simulink model "TEP_Final_NoScript"  (R2024a)
settings: Solver=FixedStepAuto  StartTime=0.0  StopTime=10  FixedStep=1/3600  RelTol=1e-3
model workspace (MAT data in the model file):
  AD : Simulink.Parameter (value not decoded)
  AG : Simulink.Parameter (value not decoded)
  AH : Simulink.Parameter (value not decoded)
  AV : Simulink.Parameter (value not decoded)
  AVP : Simulink.Parameter (value not decoded)
  BCHL : Simulink.Parameter (value not decoded)
  BCHV : Simulink.Parameter (value not decoded)
  BD : Simulink.Parameter (value not decoded)
  BG : Simulink.Parameter (value not decoded)
  BH : Simulink.Parameter (value not decoded)
  BVP : Simulink.Parameter (value not decoded)
  CD : Simulink.Parameter (value not decoded)
  CG : Simulink.Parameter (value not decoded)
  CH : Simulink.Parameter (value not decoded)
  CVP : Simulink.Parameter (value not decoded)
  XMW : Simulink.Parameter (value not decoded)
  XNS : Simulink.Parameter (value not decoded)
  XNSE : Simulink.Parameter (value not decoded)
symbols that are objects in the model workspace (value not decoded): AD, AG, AH, AV, AVP, BD, BG, BH, BVP, CD, CG, CH, CVP, XMW, XNS, XNSE
undefined symbols (not defined in the file or in its folder): magnitude, msgbox, SETPT, XMEAS, XMV
libraries: mylib x360, dspindex x28
(part 4 of 14)

== system TEP_Final_NoScript/Subsystem1/A feed stream ==
  Stream 3 : Inport
  Bus Creator : BusCreator  Inputs=4
  Bus Selector : BusSelector  OutputSignals=XMNSE(5),XMNSE(6)
  Bus Selector1 : BusSelector  OutputSignals=TST(3),XST(I;3)
  Bus Selector2 : BusSelector  OutputSignals=Stream 3
  Bus Selector3 : BusSelector  OutputSignals=signal1.XMEAS(1)
  Composition measurement mol% : Subsystem
  Constant : Constant  Value=1000
  Flow measurement in kg/h : Subsystem
  Pressure measurement in kPa : Subsystem
  Temperature measurement in C : Subsystem
  SMEAS 3 : Outport
  tag scope: SM3=global
  wires:
  Bus Selector1/1 -> Temperature measurement in C/1(T in celsius)  "<TST(3)>"
  Temperature measurement in C/1(SMEAST) -> Bus Creator/1
  [XMNSE] -> Bus Selector/1
  Bus Selector/1 -> Temperature measurement in C/2(XMNSE)  "<XMNSE(5)>"
  Bus Selector/2 -> Pressure measurement in kPa/2(XMNSE)  "<XMNSE(6)>"
  Stream 3/1 -> Bus Selector1/1
  Bus Selector1/2 -> Flow measurement in kg/h/2(XST), Composition measurement mol%/1(XST)  "<XST(I;3)>"
  Constant/1 -> Pressure measurement in kPa/1("P in mm Hg ")
  Pressure measurement in kPa/1(SMEASP) -> Bus Creator/2
  Flow measurement in kg/h/1("SMEASF ") -> Bus Creator/3  "SMEASF"
  Composition measurement mol%/1(SMEASX) -> Bus Creator/4
  Bus Creator/1 -> [SM3], SMEAS 3/1
  [XMNSE2] -> Bus Selector2/1
  Bus Selector2/1 -> Composition measurement mol%/2(XMNSE)  "<Stream 3>"
  [XMEAS] -> Bus Selector3/1
  Bus Selector3/1 -> Flow measurement in kg/h/1(XMEAS in kscmh)  "<XMEAS(1)>"

== system TEP_Final_NoScript/Subsystem1/CCIn ==
  Bus Creator : BusCreator  Inputs=3
  Bus Selector : BusSelector  OutputSignals=XMNSE(20),XMNSE(21),XMNSE(22)
  Flow measurement in kg/h : Subsystem
  Pressure measurement in kPa : Subsystem
  Temperature measurement in C : Subsystem
  SMEASCCWin : Outport
  tag scope: SMCC1=global
  wires:
  [TCWS] -> Pressure measurement in kPa/2(TC), Temperature measurement in C/1(T in celsius)
  Bus Creator/1 -> [SMCC1], SMEASCCWin/1
  [FWS] -> Flow measurement in kg/h/2(F in gpm)
  [XMNSE] -> Bus Selector/1
  Bus Selector/1 -> Temperature measurement in C/2(XMNSE)  "<XMNSE(20)>"
  Bus Selector/2 -> Pressure measurement in kPa/1(XMNSE)  "<XMNSE(21)>"
  Bus Selector/3 -> Flow measurement in kg/h/1(XMNSE)  "<XMNSE(22)>"
  Temperature measurement in C/1(SMEAST) -> Bus Creator/1
  Pressure measurement in kPa/1(SMEASP) -> Bus Creator/2
  Flow measurement in kg/h/1("SMEASF ") -> Bus Creator/3

== system TEP_Final_NoScript/Subsystem1/CCOut ==
  Bus Creator : BusCreator  Inputs=2
  Bus Selector : BusSelector  OutputSignals=XMNSE(23),XMNSE(24)
  Pressure measurement in kPa : Subsystem
  Temperature measurement in C : Subsystem
  SMEASCCWout : Outport
  tag scope: SMCC2=global
  wires:
  [TWS] -> Pressure measurement in kPa/2(TC), Temperature measurement in C/1(T in celsius)
  Bus Creator/1 -> [SMCC2], SMEASCCWout/1
  [XMNSE] -> Bus Selector/1
  Bus Selector/1 -> Temperature measurement in C/2(XMNSE)  "<XMNSE(23)>"
  Bus Selector/2 -> Pressure measurement in kPa/1(XMNSE)  "<XMNSE(24)>"
  Temperature measurement in C/1(SMEAST) -> Bus Creator/1
  Pressure measurement in kPa/1(SMEASP) -> Bus Creator/2

== system TEP_Final_NoScript/Subsystem1/CCin ==
  SMEAS : Inport
  Bus Selector : BusSelector  OutputSignals=SMEAST,SMEASP,SMEASF
  Subsystem : Subsystem
  Subsystem1 : Subsystem
  Subsystem3 : Subsystem
  tag scope: BMCC1=global, QS1=global
  wires:
  Bus Selector/1 -> Subsystem1/1(T), Subsystem3/1(TC)  "<SMEAST>"
  Subsystem/1(Bphm J/s) -> [BMCC1]  "BphmCC1"
  Subsystem3/1(Bph) -> Subsystem/1(Bph)  "BphRC1"
  Bus Selector/3 -> Subsystem1/2(F), Subsystem/2(FWR in kg/h)  "<SMEASF>"
  Subsystem1/1(Q J/s) -> [QS1]
  Bus Selector/2 -> Subsystem3/2(P)  "<SMEASP>"
  SMEAS/1 -> Bus Selector/1

== system TEP_Final_NoScript/Subsystem1/CCout ==
  SMEAS : Inport
  SMEAS1 : Inport  Port=2
  Bus Selector : BusSelector  OutputSignals=SMEAST,SMEASP
  Bus Selector1 : BusSelector  OutputSignals=SMEASF
  Subsystem : Subsystem
  Subsystem1 : Subsystem
  Subsystem3 : Subsystem
  tag scope: BMCC2=global, QS2=global
  wires:
  Bus Selector/1 -> Subsystem3/1(TC), Subsystem1/1(T)  "<SMEAST>"
  Subsystem/1(Bphm J/s) -> [BMCC2]  "BphmCC2"
  Subsystem3/1(Bph) -> Subsystem/1(Bph)  "BphRC1"
  Bus Selector1/1 -> Subsystem1/2(F), Subsystem/2(FWR in kg/h)  "<SMEASF>"
  Subsystem1/1(Q J/s) -> [QS2]
  Bus Selector/2 -> Subsystem3/2(P)  "<SMEASP>"
  SMEAS/1 -> Bus Selector/1
  SMEAS1/1 -> Bus Selector1/1

== system TEP_Final_NoScript/Subsystem1/D feed stream ==
  Stream 1 : Inport
  Bus Creator : BusCreator  Inputs=4
  Bus Selector : BusSelector  OutputSignals=XMNSE(1),XMNSE(2)
  Bus Selector1 : BusSelector  OutputSignals=TST(1),XST(I;1)
  Bus Selector2 : BusSelector  OutputSignals=Stream 1
  Bus Selector3 : BusSelector  OutputSignals=signal1.XMEAS(2)
  Composition measurement mol% : Subsystem
  Constant : Constant  Value=1000
  Flow measurement in kg/h : Subsystem
  Pressure measurement in kPa : Subsystem
  Temperature measurement in C : Subsystem
  SMEAS 1 : Outport
  tag scope: SM1=global
  wires:
  Bus Selector1/1 -> Temperature measurement in C/1(T in celsius)  "<TST(1)>"
  Temperature measurement in C/1(SMEAST) -> Bus Creator/1
  [XMNSE] -> Bus Selector/1
  Bus Selector/1 -> Temperature measurement in C/2(XMNSE)  "<XMNSE(1)>"
  Bus Selector/2 -> Pressure measurement in kPa/2(XMNSE)  "<XMNSE(2)>"
  Stream 1/1 -> Bus Selector1/1
  Bus Selector1/2 -> Composition measurement mol%/1(XST)  "<XST(I;1)>"
  Constant/1 -> Pressure measurement in kPa/1("P in mm Hg ")
  Pressure measurement in kPa/1(SMEASP) -> Bus Creator/2
  Flow measurement in kg/h/1("SMEASF ") -> Bus Creator/3  "SMEASF"
  Composition measurement mol%/1(SMEASX) -> Bus Creator/4
  Bus Creator/1 -> [SM1], SMEAS 1/1
  [XMNSE2] -> Bus Selector2/1
  Bus Selector2/1 -> Composition measurement mol%/2(XMNSE)  "<Stream 1>"
  [XMEAS] -> Bus Selector3/1
  Bus Selector3/1 -> Flow measurement in kg/h/1(XMEAS in kg/h)  "<XMEAS(2)>"

== system TEP_Final_NoScript/Subsystem1/E feed stream ==
  Stream 2 : Inport
  Bus Creator : BusCreator  Inputs=4
  Bus Selector : BusSelector  OutputSignals=XMNSE(3),XMNSE(4)
  Bus Selector1 : BusSelector  OutputSignals=TST(2),XST(I;2)
  Bus Selector2 : BusSelector  OutputSignals=Stream 2
  Bus Selector3 : BusSelector  OutputSignals=signal1.XMEAS(3)
  Composition measurement mol% : Subsystem
  Constant : Constant  Value=1000
  Flow measurement in kg/h : Subsystem
  Pressure measurement in kPa : Subsystem
  Temperature measurement in C : Subsystem
  SMEAS 2 : Outport
  tag scope: SM2=global
  wires:
  Bus Selector1/1 -> Temperature measurement in C/1(T in celsius)  "<TST(2)>"
  Temperature measurement in C/1(SMEAST) -> Bus Creator/1
  [XMNSE] -> Bus Selector/1
  Bus Selector/1 -> Temperature measurement in C/2(XMNSE)  "<XMNSE(3)>"
  Bus Selector/2 -> Pressure measurement in kPa/2(XMNSE)  "<XMNSE(4)>"
  Stream 2/1 -> Bus Selector1/1
  Bus Selector1/2 -> Composition measurement mol%/1(XST)  "<XST(I;2)>"
  Constant/1 -> Pressure measurement in kPa/1("P in mm Hg ")
  Pressure measurement in kPa/1(SMEASP) -> Bus Creator/2
  Flow measurement in kg/h/1("SMEASF ") -> Bus Creator/3  "SMEASF"
  Composition measurement mol%/1(SMEASX) -> Bus Creator/4
  Bus Creator/1 -> [SM2], SMEAS 2/1
  [XMNSE2] -> Bus Selector2/1
  Bus Selector2/1 -> Composition measurement mol%/2(XMNSE)  "<Stream 2>"
  [XMEAS] -> Bus Selector3/1
  Bus Selector3/1 -> Flow measurement in kg/h/1(XMEAS in kg/h)  "<XMEAS(3)>"

== system TEP_Final_NoScript/Subsystem1/Product stream ==
  Stream 13 : Inport
  Bus Creator : BusCreator  Inputs=4
  Bus Selector : BusSelector  OutputSignals=XMNSE(14)
  Bus Selector1 : BusSelector  OutputSignals=PTC,XST(I;13)
  Bus Selector2 : BusSelector  OutputSignals=Stream 13
  Bus Selector3 : BusSelector  OutputSignals=signal4.XMEAS(18),signal4.XMEAS(17)
  Bus Selector4 : BusSelector  OutputSignals=Stream 13
  Composition measurement mol% : Subsystem
  Flow measurement in kg/h : Subsystem
  Pressure measurement in kPa : Subsystem
  Temperature measurement in C : Subsystem
  SMEAS 13 : Outport
  tag scope: SM13=global
  wires:
  Temperature measurement in C/1(SMEAST) -> Bus Creator/1
  [XMNSE] -> Bus Selector/1
  Stream 13/1 -> Bus Selector1/1
  Pressure measurement in kPa/1(SMEASP) -> Bus Creator/2
  Flow measurement in kg/h/1("SMEASF ") -> Bus Creator/3  "SMEASF"
  Composition measurement mol%/1(SMEASX) -> Bus Creator/4
  Bus Creator/1 -> [SM13], SMEAS 13/1
  [XMNSE2] -> Bus Selector2/1
  Bus Selector2/1 -> Composition measurement mol%/2(XMNSE2)  "<Stream 13>"
  [XMEAS] -> Bus Selector3/1
  Bus Selector/1 -> Pressure measurement in kPa/2(XMNSE)  "<XMNSE(14)>"
  Bus Selector1/1 -> Pressure measurement in kPa/1("P in mm Hg ")  "<PTC>"
  Bus Selector3/1 -> Temperature measurement in C/1(XMEAS in celsius)  "<XMEAS(18)>"
  Bus Selector3/2 -> Flow measurement in kg/h/1(XMEAS in m^3/h)  "<XMEAS(17)>"
  Bus Selector1/2 -> Composition measurement mol%/1(XST), Flow measurement in kg/h/2(XST)  "<XST(I;13)>"
  [XMNSE3] -> Bus Selector4/1
  Bus Selector4/1 -> Composition measurement mol%/3(XMNSE3)  "<Stream 13>"

== system TEP_Final_NoScript/Subsystem1/Purge stream ==
  Stream 10 : Inport
  Bus Creator : BusCreator  Inputs=4
  Bus Selector1 : BusSelector  OutputSignals=signal1.XST(I;10)
  Bus Selector3 : BusSelector  OutputSignals=signal3.XMEAS(11),signal3.XMEAS(13),signal3.XMEAS(10),signal9
  Composition measurement mol% : Subsystem
  Flow measurement in kg/h : Subsystem
  Pressure measurement in kPa : Subsystem
  Temperature measurement in C : Subsystem
  SMEAS 10 : Outport
  tag scope: SM10=global
  wires:
  Temperature measurement in C/1(SMEAST) -> Bus Creator/1  "SMEAST"
  Stream 10/1 -> Bus Selector1/1
  Bus Selector1/1 -> Flow measurement in kg/h/2(XST)  "<XST(I;10)>"
  Pressure measurement in kPa/1(SMEASP) -> Bus Creator/2
  Flow measurement in kg/h/1("SMEASF ") -> Bus Creator/3  "SMEASF"
  Composition measurement mol%/1(SMEASX) -> Bus Creator/4
  Bus Creator/1 -> [SM10], SMEAS 10/1
  [XMEAS] -> Bus Selector3/1
  Bus Selector3/1 -> Temperature measurement in C/1(XMEAS in celsius)  "<XMEAS(11)>"
  Bus Selector3/2 -> Pressure measurement in kPa/1(XMEAS in kPa gauge)  "<XMEAS(13)>"
  Bus Selector3/3 -> Flow measurement in kg/h/1(XMEAS in kscmh)  "<XMEAS(10)>"
  Bus Selector3/4 -> Composition measurement mol%/1(XMEAS)  "<signal9>"

== system TEP_Final_NoScript/Subsystem1/RCIn ==
  Bus Creator : BusCreator  Inputs=3
  Bus Selector : BusSelector  OutputSignals=XMNSE(15),XMNSE(16),XMNSE(17)
  Flow measurement in kg/h : Subsystem
  Pressure measurement in kPa : Subsystem
  Temperature measurement in C : Subsystem
  SMEASRCWin : Outport
  tag scope: SMRC1=global
  wires:
  [TCWR] -> Pressure measurement in kPa/2(TC), Temperature measurement in C/1(T in celsius)
  [FWR] -> Flow measurement in kg/h/2(F in gpm)
  [XMNSE] -> Bus Selector/1
  Bus Selector/1 -> Temperature measurement in C/2(XMNSE)  "<XMNSE(15)>"
  Bus Selector/2 -> Pressure measurement in kPa/1(XMNSE)  "<XMNSE(16)>"
  Bus Selector/3 -> Flow measurement in kg/h/1(XMNSE)  "<XMNSE(17)>"
  Temperature measurement in C/1(SMEAST) -> Bus Creator/1
  Pressure measurement in kPa/1(SMEASP) -> Bus Creator/2
  Flow measurement in kg/h/1("SMEASF ") -> Bus Creator/3
  Bus Creator/1 -> [SMRC1], SMEASRCWin/1

== system TEP_Final_NoScript/Subsystem1/RCOut ==
  Bus Creator : BusCreator  Inputs=2
  Bus Selector : BusSelector  OutputSignals=XMNSE(18),XMNSE(19)
  Pressure measurement in kPa : Subsystem
  Temperature measurement in C : Subsystem
  SMEASRCWout : Outport
  tag scope: SMRC2=global
  wires:
  [TWR] -> Pressure measurement in kPa/2(TC), Temperature measurement in C/1(T in celsius)
  Bus Creator/1 -> [SMRC2], SMEASRCWout/1
  [XMNSE] -> Bus Selector/1
  Bus Selector/1 -> Temperature measurement in C/2(XMNSE)  "<XMNSE(18)>"
  Bus Selector/2 -> Pressure measurement in kPa/1(XMNSE)  "<XMNSE(19)>"
  Temperature measurement in C/1(SMEAST) -> Bus Creator/1
  Pressure measurement in kPa/1(SMEASP) -> Bus Creator/2

== system TEP_Final_NoScript/Subsystem1/RCin ==
  SMEAS : Inport
  Bus Selector : BusSelector  OutputSignals=SMEAST,SMEASP,SMEASF
  Subsystem : Subsystem
  Subsystem1 : Subsystem
  Subsystem3 : Subsystem
  tag scope: BMRC1=global, QR1=global
  wires:
  Bus Selector/1 -> Subsystem1/1(T), Subsystem3/1(TC)  "<SMEAST>"
  Subsystem/1(Bphm J/s) -> [BMRC1]  "BphmRC1"
  Subsystem3/1(Bph) -> Subsystem/1(Bph)  "BphRC1"
  Bus Selector/3 -> Subsystem1/2(F), Subsystem/2(FWR in kg/h)  "<SMEASF>"
  Subsystem1/1(Q J/s) -> [QR1]
  Bus Selector/2 -> Subsystem3/2(P)  "<SMEASP>"
  SMEAS/1 -> Bus Selector/1

== system TEP_Final_NoScript/Subsystem1/RCout ==
  SMEAS : Inport
  SMEAS1 : Inport  Port=2
  Bus Selector : BusSelector  OutputSignals=SMEAST,SMEASP
  Bus Selector1 : BusSelector  OutputSignals=SMEASF
  Subsystem : Subsystem
  Subsystem1 : Subsystem
  Subsystem3 : Subsystem
  tag scope: BMRC2=global, QR2=global
  wires:
  Bus Selector/1 -> Subsystem3/1(TC), Subsystem1/1(T)  "<SMEAST>"
  Subsystem/1(Bphm J/s) -> [BMRC2]  "BphmRC2"
  Subsystem3/1(Bph) -> Subsystem/1(Bph)  "BphRC1"
  Bus Selector1/1 -> Subsystem1/2(F), Subsystem/2(FWR in kg/h)  "<SMEASF>"
  Subsystem1/1(Q J/s) -> [QR2]
  Bus Selector/2 -> Subsystem3/2(P)  "<SMEASP>"
  SMEAS/1 -> Bus Selector/1
  SMEAS1/1 -> Bus Selector1/1

== system TEP_Final_NoScript/Subsystem1/Reactor feed stream ==
  Stream 6 : Inport
  Bus Creator : BusCreator  Inputs=4
  Bus Selector : BusSelector  OutputSignals=XMNSE(11)
  Bus Selector1 : BusSelector  OutputSignals=signal1.TST(6) = TST(7),signal1.XST(I;6) = XST(I;7)
  Bus Selector2 : BusSelector  OutputSignals=Stream 6
  Bus Selector3 : BusSelector  OutputSignals=signal4.XMEAS(16),signal2.XMEAS(6),signal8
  Composition measurement mol% : Subsystem
  Flow measurement in kg/h : Subsystem
  Pressure measurement in kPa : Subsystem
  Temperature measurement in C : Subsystem
  SMEAS 6 : Outport
  tag scope: SM6=global
  wires:
  Bus Selector1/1 -> Temperature measurement in C/1(T in celsius)  "<TST(6) = TST(7)>"
  Temperature measurement in C/1(SMEAST) -> Bus Creator/1
  [XMNSE] -> Bus Selector/1
  Bus Selector/1 -> Temperature measurement in C/2(XMNSE)  "<XMNSE(11)>"
  Stream 6/1 -> Bus Selector1/1
  Bus Selector1/2 -> Flow measurement in kg/h/2(XST), Composition measurement mol%/1(XST)  "<XST(I;6) = XST(I;7)>"
  [XMEAS] -> Bus Selector3/1
  Pressure measurement in kPa/1(SMEASP) -> Bus Creator/2
  Flow measurement in kg/h/1("SMEASF ") -> Bus Creator/3  "SMEASF"
  Composition measurement mol%/1(SMEASX) -> Bus Creator/4
  Bus Creator/1 -> [SM6], SMEAS 6/1
  [XMNSE2] -> Bus Selector2/1
  Bus Selector2/1 -> Composition measurement mol%/2(XMNSE)  "<Stream 6>"
  Bus Selector3/1 -> Pressure measurement in kPa/1(XMEAS in kPa gauge)  "<XMEAS(16)>"
  Bus Selector3/2 -> Flow measurement in kg/h/1(XMEAS in kscmh)  "<XMEAS(6)>"
  Bus Selector3/3 -> Composition measurement mol%/3(XMEAS)  "<signal8>"

== system TEP_Final_NoScript/Subsystem1/Reactor product stream ==
  Stream 8 : Inport
  Bus Creator : BusCreator  Inputs=4
  Bus Selector : BusSelector  OutputSignals=XMNSE(12)
  Bus Selector1 : BusSelector  OutputSignals=signal1.XST(I;8),signal1.FTM(8)
  Bus Selector2 : BusSelector  OutputSignals=Stream 8
  Bus Selector3 : BusSelector  OutputSignals=signal2.XMEAS(9),signal2.XMEAS(7)
  Composition measurement mol% : Subsystem
  Flow measurement in kg/h : Subsystem
  Pressure measurement in kPa : Subsystem
  Temperature measurement in C : Subsystem
  SMEAS 8 : Outport
  tag scope: SM8=global
  wires:
  Temperature measurement in C/1(SMEAST) -> Bus Creator/1
  [XMNSE] -> Bus Selector/1
  Stream 8/1 -> Bus Selector1/1
  Bus Selector1/1 -> Composition measurement mol%/1(XST), Flow measurement in kg/h/1(XST)  "<XST(I;8)>"
  Pressure measurement in kPa/1(SMEASP) -> Bus Creator/2
  Flow measurement in kg/h/1("SMEASF ") -> Bus Creator/3
  Composition measurement mol%/1(SMEASX) -> Bus Creator/4
  Bus Creator/1 -> [SM8], SMEAS 8/1
  [XMNSE2] -> Bus Selector2/1
  Bus Selector2/1 -> Composition measurement mol%/2(XMNSE)  "<Stream 8>"
  [XMEAS] -> Bus Selector3/1
  Bus Selector3/1 -> Temperature measurement in C/1(XMEAS in celsius)  "<XMEAS(9)>"
  Bus Selector3/2 -> Pressure measurement in kPa/1(XMEAS in kPa gauge)  "<XMEAS(7)>"
  Bus Selector1/2 -> Flow measurement in kg/h/3(F in lb-mol/h)  "<FTM(8)>"
  Bus Selector/1 -> Flow measurement in kg/h/2(XMNSE)  "<XMNSE(12)>"

== system TEP_Final_NoScript/Subsystem1/Separator recycle stream ==
  Stream 9 : Inport
  Bus Creator : BusCreator  Inputs=4
  Bus Selector1 : BusSelector  OutputSignals=signal2.XST(I;9)
  Bus Selector2 : BusSelector  OutputSignals=Stream 9
  Bus Selector3 : BusSelector  OutputSignals=signal3.XMEAS(11),signal3.XMEAS(13),signal1.XMEAS(5)
  Composition measurement mol% : Subsystem
  Flow measurement in kg/h : Subsystem
  Pressure measurement in kPa : Subsystem
  Temperature measurement in C : Subsystem
  SMEAS 9 : Outport
  tag scope: SM9=global
  wires:
  Temperature measurement in C/1(SMEAST) -> Bus Creator/1  "SMEAST"
  Stream 9/1 -> Bus Selector1/1
  Bus Selector1/1 -> Flow measurement in kg/h/2(XST), Composition measurement mol%/1(XST)  "<XST(I;9)>"
  Pressure measurement in kPa/1(SMEASP) -> Bus Creator/2
  Flow measurement in kg/h/1("SMEASF ") -> Bus Creator/3  "SMEASF"
  Composition measurement mol%/1(SMEASX) -> Bus Creator/4
  Bus Creator/1 -> [SM9], SMEAS 9/1
  [XMNSE2] -> Bus Selector2/1
  Bus Selector2/1 -> Composition measurement mol%/2(XMNSE)  "<Stream 9>"
  [XMEAS] -> Bus Selector3/1
  Bus Selector3/1 -> Temperature measurement in C/1(XMEAS in celsius)  "<XMEAS(11)>"
  Bus Selector3/2 -> Pressure measurement in kPa/1(XMEAS in kPa gauge)  "<XMEAS(13)>"
  Bus Selector3/3 -> Flow measurement in kg/h/1(XMEAS in kscmh)  "<XMEAS(5)>"

== system TEP_Final_NoScript/Subsystem1/Separator underflow stream ==
  Stream 11 : Inport
  Bus Creator : BusCreator  Inputs=4
  Bus Selector1 : BusSelector  OutputSignals=signal1.PTSL,signal1.XST(I;11)
  Bus Selector2 : BusSelector  OutputSignals=Stream 11
  Bus Selector3 : BusSelector  OutputSignals=signal3.XMEAS(11),signal3.XMEAS(14)
  Bus Selector4 : BusSelector  OutputSignals=XMNSE(13)
  Composition measurement mol% : Subsystem
  Flow measurement in kg/h : Subsystem
  Pressure measurement in kPa : Subsystem
  Temperature measurement in C : Subsystem
  SMEAS 11 : Outport
  tag scope: SM11=global
  wires:
  Temperature measurement in C/1(SMEAST) -> Bus Creator/1
  [XMNSE] -> Bus Selector4/1
  Stream 11/1 -> Bus Selector1/1
  Pressure measurement in kPa/1(SMEASP) -> Bus Creator/2
  Flow measurement in kg/h/1("SMEASF ") -> Bus Creator/3  "SMEASF"
  Composition measurement mol%/1(SMEASX) -> Bus Creator/4
  Bus Creator/1 -> [SM11], SMEAS 11/1
  [XMNSE3] -> Bus Selector2/1
  Bus Selector2/1 -> Composition measurement mol%/2(XMNSE)  "<Stream 11>"
  [XMEAS] -> Bus Selector3/1
  Bus Selector4/1 -> Pressure measurement in kPa/2(XMNSE)  "<XMNSE(13)>"
  Bus Selector1/1 -> Pressure measurement in kPa/1("P in mm Hg ")  "<PTSL>"
  Bus Selector1/2 -> Flow measurement in kg/h/2(XST), Composition measurement mol%/1(XST)  "<XST(I;11)>"
  Bus Selector3/1 -> Temperature measurement in C/1(XMEAS in celsius)  "<XMEAS(11)>"
  Bus Selector3/2 -> Flow measurement in kg/h/1(XMEAS in m^3/h)  "<XMEAS(14)>"

== system TEP_Final_NoScript/Subsystem1/Stripper recycle stream ==
  Stream 5 : Inport
  Bus Creator : BusCreator  Inputs=4
  Bus Selector : BusSelector  OutputSignals=XMNSE(9),XMNSE(10)
  Bus Selector1 : BusSelector  OutputSignals=TST(5),XST(I;5),FTM(5)
  Bus Selector2 : BusSelector  OutputSignals=Stream 5
  Bus Selector3 : BusSelector  OutputSignals=signal4.XMEAS(16)
  Composition measurement mol% : Subsystem
  Flow measurement in kg/h : Subsystem
  Pressure measurement in kPa : Subsystem
  Temperature measurement in C : Subsystem
  SMEAS 5 : Outport
  tag scope: SM5=global
  wires:
  Bus Selector1/1 -> Temperature measurement in C/1(T in celsius)  "<TST(5)>"
  Temperature measurement in C/1(SMEAST) -> Bus Creator/1
  [XMNSE] -> Bus Selector/1
  Bus Selector/1 -> Temperature measurement in C/2(XMNSE)  "<XMNSE(9)>"
  Stream 5/1 -> Bus Selector1/1
  Bus Selector1/2 -> Composition measurement mol%/1(XST), Flow measurement in kg/h/1(XST)  "<XST(I;5)>"
  [XMEAS] -> Bus Selector3/1
  Pressure measurement in kPa/1(SMEASP) -> Bus Creator/2
  Flow measurement in kg/h/1("SMEASF ") -> Bus Creator/3
  Composition measurement mol%/1(SMEASX) -> Bus Creator/4
  Bus Creator/1 -> [SM5], SMEAS 5/1
  [XMNSE2] -> Bus Selector2/1
  Bus Selector2/1 -> Composition measurement mol%/2(XMNSE)  "<Stream 5>"
  Bus Selector3/1 -> Pressure measurement in kPa/1(XMEAS in kPa gauge)  "<XMEAS(16)>"
  Bus Selector1/3 -> Flow measurement in kg/h/3(F in lb-mol/h)  "<FTM(5)>"
  Bus Selector/2 -> Flow measurement in kg/h/2(XMNSE)  "<XMNSE(10)>"

== system TEP_Final_NoScript/Subsystem1/Subsystem1 ==
  SMEAS 8 : Inport
  Bus Creator3 : BusCreator  Inputs=2
  Bus Selector1 : BusSelector  OutputSignals=SMEAST,SMEASP,SMEASF,SMEASX
  Bus Selector2 : BusSelector  OutputSignals=signal1.HST(8),signal1.Phase
  Exergy1 : mylib/Exergy  SystemSampleTime=-1  VariantActivationTime=update diagram  AllowFlexibleInterface=on  Latency=0  AutoFrameSizeCalculation=off
      settings: SourceProductName=TEP Library
  J/s : Gain  Gain=0.29307107e6
  Subsystem : mylib/Subsystem  SystemSampleTime=-1  VariantActivationTime=update diagram  AllowFlexibleInterface=on  Latency=0  AutoFrameSizeCalculation=off
      settings: SourceProductName=TEP Library
  Subsystem1 : Subsystem
  mmBtu/hr : Product
  tag scope: BM8=global, Q8=global
  wires:
  Exergy1/1 -> Subsystem/1  "Bch8"
  Exergy1/2 -> Subsystem/2  "Bph8"
  Subsystem/1 -> Bus Creator3/1  "Bchm8"
  Subsystem/2 -> Bus Creator3/2  "Bphm8"
  Bus Creator3/1 -> [BM8]  "BM8"
  mmBtu/hr/1 -> J/s/1
  J/s/1 -> [Q8]
  [PropertiesStream8] -> Bus Selector2/1
  SMEAS 8/1 -> Subsystem1/1(SMEASX)
  Subsystem1/1(SMEASXOut) -> Bus Selector1/1
  Bus Selector2/1 -> mmBtu/hr/2  "<HST(8)>"
  Bus Selector2/2 -> Exergy1/1  "<Phase>"
  Bus Selector1/1 -> Exergy1/2  "<SMEAST>"
  Bus Selector1/2 -> Exergy1/4  "<SMEASP>"
  Bus Selector1/3 -> mmBtu/hr/1, Subsystem/3  "<SMEASF>"
  Bus Selector1/4 -> Exergy1/3  "<SMEASX>"

== system TEP_Final_NoScript/Subsystem1/Subsystem10 ==
  Bus Creator : BusCreator  Inputs=15
  B : Outport  VectorParamsAs1DForOutWhenUnconnected=off
  wires:
  Bus Creator/1 -> B/1
  [BMCC1] -> Bus Creator/14
  [BM11] -> Bus Creator/10
  [BM5] -> Bus Creator/5
  [BM1] -> Bus Creator/1
  [BM6] -> Bus Creator/6
  [BM9] -> Bus Creator/8
  [BM3] -> Bus Creator/3
  [BM4] -> Bus Creator/4
  [BM10] -> Bus Creator/9
  [BMRC1] -> Bus Creator/12
  [BM2] -> Bus Creator/2
  [BM13] -> Bus Creator/11
  [BM8] -> Bus Creator/7
  [BMRC2] -> Bus Creator/13
  [BMCC2] -> Bus Creator/15

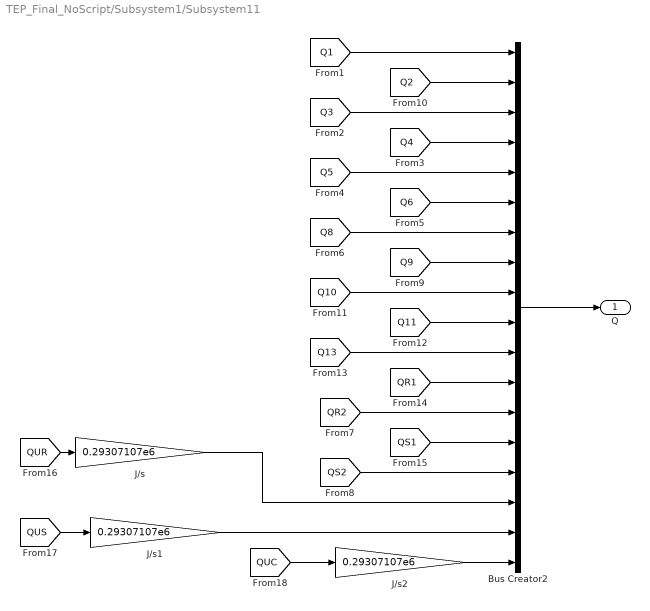
== system TEP_Final_NoScript/Subsystem1/Subsystem11 ==
  Bus Creator2 : BusCreator  Inputs=18
  J/s : Gain  Gain=0.29307107e6
  J/s1 : Gain  Gain=0.29307107e6
  J/s2 : Gain  Gain=0.29307107e6
  Q : Outport  VectorParamsAs1DForOutWhenUnconnected=off
  wires:
  [Q3] -> Bus Creator2/3
  Bus Creator2/1 -> Q/1
  [Q6] -> Bus Creator2/6
  [Q1] -> Bus Creator2/1
  [Q2] -> Bus Creator2/2
  [Q8] -> Bus Creator2/7
  [Q4] -> Bus Creator2/4
  [Q5] -> Bus Creator2/5
  [Q9] -> Bus Creator2/8
  [Q10] -> Bus Creator2/9
  [Q11] -> Bus Creator2/10
  [Q13] -> Bus Creator2/11
  [QR2] -> Bus Creator2/13
  [QR1] -> Bus Creator2/12
  [QS2] -> Bus Creator2/15
  [QS1] -> Bus Creator2/14
  [QUR] -> J/s/1
  J/s/1 -> Bus Creator2/16
  [QUS] -> J/s1/1
  J/s1/1 -> Bus Creator2/17
  [QUC] -> J/s2/1
  J/s2/1 -> Bus Creator2/18

== system TEP_Final_NoScript/Subsystem1/Subsystem13 ==
  SMEAS 6 : Inport
  Bus Creator3 : BusCreator  Inputs=2
  Bus Selector1 : BusSelector  OutputSignals=SMEAST,SMEASP,SMEASF,SMEASX
  Bus Selector2 : BusSelector  OutputSignals=signal1.HST(6) = HST(7),signal1.Phase
  Exergy1 : mylib/Exergy  SystemSampleTime=-1  VariantActivationTime=update diagram  AllowFlexibleInterface=on  Latency=0  AutoFrameSizeCalculation=off
      settings: SourceProductName=TEP Library
  J/s : Gain  Gain=0.29307107e6
  Subsystem : mylib/Subsystem  SystemSampleTime=-1  VariantActivationTime=update diagram  AllowFlexibleInterface=on  Latency=0  AutoFrameSizeCalculation=off
      settings: SourceProductName=TEP Library
  Subsystem1 : Subsystem
  mmBtu/hr : Product
  tag scope: BM6=global, Q6=global
  wires:
  Exergy1/1 -> Subsystem/1  "Bch6"
  Exergy1/2 -> Subsystem/2  "Bph6"
  Subsystem/1 -> Bus Creator3/1  "Bchm6"
  Subsystem/2 -> Bus Creator3/2  "Bphm6"
  Bus Creator3/1 -> [BM6]  "BM6"
  mmBtu/hr/1 -> J/s/1
  J/s/1 -> [Q6]
  SMEAS 6/1 -> Subsystem1/1(SMEASX)
  [PropertiesStream6] -> Bus Selector2/1
  Subsystem1/1(SMEASXOut) -> Bus Selector1/1
  Bus Selector2/1 -> mmBtu/hr/2  "<HST(6) = HST(7)>"
  Bus Selector2/2 -> Exergy1/1  "<Phase>"
  Bus Selector1/1 -> Exergy1/2  "<SMEAST>"
  Bus Selector1/2 -> Exergy1/4  "<SMEASP>"
  Bus Selector1/3 -> mmBtu/hr/1, Subsystem/3  "<SMEASF>"
  Bus Selector1/4 -> Exergy1/3  "<SMEASX>"

== system TEP_Final_NoScript/Subsystem1/Subsystem14 ==
  SMEAS 11 : Inport
  Bus Creator3 : BusCreator  Inputs=2
  Bus Selector1 : BusSelector  OutputSignals=SMEAST,SMEASP,SMEASF,SMEASX
  Bus Selector2 : BusSelector  OutputSignals=signal1.HST(11),signal1.Phase
  Exergy1 : mylib/Exergy  SystemSampleTime=-1  VariantActivationTime=update diagram  AllowFlexibleInterface=on  Latency=0  AutoFrameSizeCalculation=off
      settings: SourceProductName=TEP Library
  J/s : Gain  Gain=0.29307107e6
  Subsystem : mylib/Subsystem  SystemSampleTime=-1  VariantActivationTime=update diagram  AllowFlexibleInterface=on  Latency=0  AutoFrameSizeCalculation=off
      settings: SourceProductName=TEP Library
  Subsystem1 : Subsystem
  mmBtu/hr : Product
  tag scope: BM11=global, Q11=global
  wires:
  Exergy1/1 -> Subsystem/1  "Bch11"
  Exergy1/2 -> Subsystem/2  "Bph11"
  Subsystem/1 -> Bus Creator3/1  "Bchm11"
  Subsystem/2 -> Bus Creator3/2  "Bphm11"
  Bus Creator3/1 -> [BM11]  "BM11"
  J/s/1 -> [Q11]
  mmBtu/hr/1 -> J/s/1
  [PropertiesStream11] -> Bus Selector2/1
  SMEAS 11/1 -> Subsystem1/1(SMEASX)
  Subsystem1/1(SMEASXOut) -> Bus Selector1/1
  Bus Selector2/1 -> mmBtu/hr/2  "<HST(11)>"
  Bus Selector2/2 -> Exergy1/1  "<Phase>"
  Bus Selector1/1 -> Exergy1/2  "<SMEAST>"
  Bus Selector1/2 -> Exergy1/4  "<SMEASP>"
  Bus Selector1/3 -> Subsystem/3, mmBtu/hr/1  "<SMEASF>"
  Bus Selector1/4 -> Exergy1/3  "<SMEASX>"

== system TEP_Final_NoScript/Subsystem1/Subsystem15 ==
  SMEAS 2 : Inport
  Bus Creator3 : BusCreator  Inputs=2
  Bus Selector1 : BusSelector  OutputSignals=SMEAST,SMEASP,SMEASF,SMEASX
  Bus Selector2 : BusSelector  OutputSignals=HST(2)
  Exergy1 : mylib/Exergy  SystemSampleTime=-1  VariantActivationTime=update diagram  AllowFlexibleInterface=on  Latency=0  AutoFrameSizeCalculation=off
      settings: SourceProductName=TEP Library
  ITY : Constant
  J/s : Gain  Gain=0.29307107e6
  Subsystem : mylib/Subsystem  SystemSampleTime=-1  VariantActivationTime=update diagram  AllowFlexibleInterface=on  Latency=0  AutoFrameSizeCalculation=off
      settings: SourceProductName=TEP Library
  Subsystem1 : Subsystem
  mmBtu/hr : Product
  tag scope: BM2=global, Q2=global
  wires:
  Exergy1/1 -> Subsystem/1  "Bch2"
  Exergy1/2 -> Subsystem/2  "Bph2"
  Subsystem/1 -> Bus Creator3/1  "Bchm2"
  Subsystem/2 -> Bus Creator3/2  "Bphm2"
  Bus Creator3/1 -> [BM2]  "BM2"
  ITY/1 -> Exergy1/1
  mmBtu/hr/1 -> J/s/1
  J/s/1 -> [Q2]
  SMEAS 2/1 -> Subsystem1/1(SMEASX)
  Subsystem1/1(SMEASXOut) -> Bus Selector1/1
  Bus Selector1/1 -> Exergy1/2  "<SMEAST>"
  Bus Selector1/2 -> Exergy1/4  "<SMEASP>"
  Bus Selector1/3 -> Subsystem/3, mmBtu/hr/1  "<SMEASF>"
  Bus Selector1/4 -> Exergy1/3  "<SMEASX>"
  [PropertiesStream2] -> Bus Selector2/1
  Bus Selector2/1 -> mmBtu/hr/2  "<HST(2)>"

== system TEP_Final_NoScript/Subsystem1/Subsystem16 ==
  SMEAS 3 : Inport
  Bus Creator3 : BusCreator  Inputs=2
  Bus Selector1 : BusSelector  OutputSignals=SMEAST,SMEASP,SMEASF,SMEASX
  Bus Selector2 : BusSelector  OutputSignals=HST(3)
  Exergy1 : mylib/Exergy  SystemSampleTime=-1  VariantActivationTime=update diagram  AllowFlexibleInterface=on  Latency=0  AutoFrameSizeCalculation=off
      settings: SourceProductName=TEP Library
  ITY : Constant
  J/s : Gain  Gain=0.29307107e6
  Subsystem : mylib/Subsystem  SystemSampleTime=-1  VariantActivationTime=update diagram  AllowFlexibleInterface=on  Latency=0  AutoFrameSizeCalculation=off
      settings: SourceProductName=TEP Library
  Subsystem1 : Subsystem
  mmBtu/hr : Product
  tag scope: BM3=global, Q3=global
  wires:
  Exergy1/1 -> Subsystem/1  "Bch3"
  Exergy1/2 -> Subsystem/2  "Bph3"
  Subsystem/1 -> Bus Creator3/1  "Bchm3"
  Subsystem/2 -> Bus Creator3/2  "Bphm3"
  Bus Creator3/1 -> [BM3]  "BM3"
  ITY/1 -> Exergy1/1
  mmBtu/hr/1 -> J/s/1
  J/s/1 -> [Q3]
  Subsystem1/1(SMEASXOut) -> Bus Selector1/1
  SMEAS 3/1 -> Subsystem1/1(SMEASX)
  [PropertiesStream3] -> Bus Selector2/1
  Bus Selector2/1 -> mmBtu/hr/2  "<HST(3)>"
  Bus Selector1/1 -> Exergy1/2  "<SMEAST>"
  Bus Selector1/2 -> Exergy1/4  "<SMEASP>"
  Bus Selector1/3 -> Subsystem/3, mmBtu/hr/1  "<SMEASF>"
  Bus Selector1/4 -> Exergy1/3  "<SMEASX>"

== system TEP_Final_NoScript/Subsystem1/Subsystem17 ==
  SMEAS 4 : Inport
  Bus Creator3 : BusCreator  Inputs=2
  Bus Selector1 : BusSelector  OutputSignals=SMEAST,SMEASP,SMEASF,SMEASX
  Bus Selector2 : BusSelector  OutputSignals=HST(4)
  Exergy1 : mylib/Exergy  SystemSampleTime=-1  VariantActivationTime=update diagram  AllowFlexibleInterface=on  Latency=0  AutoFrameSizeCalculation=off
      settings: SourceProductName=TEP Library
  ITY : Constant
  J/s : Gain  Gain=0.29307107e6
  Subsystem : mylib/Subsystem  SystemSampleTime=-1  VariantActivationTime=update diagram  AllowFlexibleInterface=on  Latency=0  AutoFrameSizeCalculation=off
      settings: SourceProductName=TEP Library
  Subsystem1 : Subsystem
  mmBtu/hr : Product
  tag scope: BM4=global, Q4=global
  wires:
  Exergy1/1 -> Subsystem/1  "Bch4"
  Exergy1/2 -> Subsystem/2  "Bph4"
  Subsystem/1 -> Bus Creator3/1  "Bchm4"
  Subsystem/2 -> Bus Creator3/2  "Bphm4"
  Bus Creator3/1 -> [BM4]  "BM4"
  ITY/1 -> Exergy1/1
  mmBtu/hr/1 -> J/s/1
  J/s/1 -> [Q4]
  SMEAS 4/1 -> Subsystem1/1(SMEASX)
  [PropertiesStream4] -> Bus Selector2/1
  Subsystem1/1(SMEASXOut) -> Bus Selector1/1
  Bus Selector1/1 -> Exergy1/2  "<SMEAST>"
  Bus Selector1/2 -> Exergy1/4  "<SMEASP>"
  Bus Selector1/3 -> mmBtu/hr/1, Subsystem/3  "<SMEASF>"
  Bus Selector1/4 -> Exergy1/3  "<SMEASX>"
  Bus Selector2/1 -> mmBtu/hr/2  "<HST(4)>"

== system TEP_Final_NoScript/Subsystem1/Subsystem2 ==
  SMEAS 9 : Inport
  Bus Creator3 : BusCreator  Inputs=2
  Bus Selector1 : BusSelector  OutputSignals=SMEAST,SMEASP,SMEASF,SMEASX
  Bus Selector2 : BusSelector  OutputSignals=signal2.HST(9),signal2.Phase
  Exergy1 : mylib/Exergy  SystemSampleTime=-1  VariantActivationTime=update diagram  AllowFlexibleInterface=on  Latency=0  AutoFrameSizeCalculation=off
      settings: SourceProductName=TEP Library
  J/s : Gain  Gain=0.29307107e6
  Subsystem : mylib/Subsystem  SystemSampleTime=-1  VariantActivationTime=update diagram  AllowFlexibleInterface=on  Latency=0  AutoFrameSizeCalculation=off
      settings: SourceProductName=TEP Library
  Subsystem1 : Subsystem
  mmBtu/hr : Product
  tag scope: BM9=global, Q9=global
  wires:
  Exergy1/1 -> Subsystem/1  "Bch9"
  Exergy1/2 -> Subsystem/2  "Bph9"
  Subsystem/1 -> Bus Creator3/1  "Bchm9"
  Subsystem/2 -> Bus Creator3/2  "Bphm9"
  Bus Creator3/1 -> [BM9]  "BM9"
  mmBtu/hr/1 -> J/s/1
  J/s/1 -> [Q9]
  [PropertiesStream9] -> Bus Selector2/1
  SMEAS 9/1 -> Subsystem1/1(SMEASX)
  Subsystem1/1(SMEASXOut) -> Bus Selector1/1
  Bus Selector2/1 -> mmBtu/hr/2  "<HST(9)>"
  Bus Selector2/2 -> Exergy1/1  "<Phase>"
  Bus Selector1/1 -> Exergy1/2  "<SMEAST>"
  Bus Selector1/2 -> Exergy1/4  "<SMEASP>"
  Bus Selector1/3 -> mmBtu/hr/1, Subsystem/3  "<SMEASF>"
  Bus Selector1/4 -> Exergy1/3  "<SMEASX>"

== system TEP_Final_NoScript/Subsystem1/Subsystem3 ==
  SMEAS 10 : Inport
  Bus Creator3 : BusCreator  Inputs=2
  Bus Selector1 : BusSelector  OutputSignals=SMEAST,SMEASP,SMEASF,SMEASX
  Bus Selector2 : BusSelector  OutputSignals=signal1.HST(10),signal1.Phase
  Exergy1 : mylib/Exergy  SystemSampleTime=-1  VariantActivationTime=update diagram  AllowFlexibleInterface=on  Latency=0  AutoFrameSizeCalculation=off
      settings: SourceProductName=TEP Library
  J/s : Gain  Gain=0.29307107e6
  Subsystem : mylib/Subsystem  SystemSampleTime=-1  VariantActivationTime=update diagram  AllowFlexibleInterface=on  Latency=0  AutoFrameSizeCalculation=off
      settings: SourceProductName=TEP Library
  Subsystem1 : Subsystem
  mmBtu/hr : Product
  tag scope: BM10=global, Q10=global
  wires:
  Exergy1/1 -> Subsystem/1  "Bch10"
  Exergy1/2 -> Subsystem/2  "Bph10"
  Subsystem/1 -> Bus Creator3/1  "Bchm10"
  Subsystem/2 -> Bus Creator3/2  "Bphm10"
  Bus Creator3/1 -> [BM10]  "BM10"
  mmBtu/hr/1 -> J/s/1
  J/s/1 -> [Q10]
  [PropertiesStream10] -> Bus Selector2/1
  SMEAS 10/1 -> Subsystem1/1(SMEASX)
  Subsystem1/1(SMEASXOut) -> Bus Selector1/1
  Bus Selector2/1 -> mmBtu/hr/2  "<HST(10)>"
  Bus Selector2/2 -> Exergy1/1  "<Phase>"
  Bus Selector1/1 -> Exergy1/2  "<SMEAST>"
  Bus Selector1/2 -> Exergy1/4  "<SMEASP>"
  Bus Selector1/3 -> mmBtu/hr/1, Subsystem/3  "<SMEASF>"
  Bus Selector1/4 -> Exergy1/3  "<SMEASX>"

== system TEP_Final_NoScript/Subsystem1/Subsystem4 ==
  SMEAS 5 : Inport
  Bus Creator3 : BusCreator  Inputs=2
  Bus Selector1 : BusSelector  OutputSignals=SMEAST,SMEASP,SMEASF,SMEASX
  Bus Selector2 : BusSelector  OutputSignals=HST(5),Phase
  Exergy1 : mylib/Exergy  SystemSampleTime=-1  VariantActivationTime=update diagram  AllowFlexibleInterface=on  Latency=0  AutoFrameSizeCalculation=off
      settings: SourceProductName=TEP Library
  J/s : Gain  Gain=0.29307107e6
  Subsystem : mylib/Subsystem  SystemSampleTime=-1  VariantActivationTime=update diagram  AllowFlexibleInterface=on  Latency=0  AutoFrameSizeCalculation=off
      settings: SourceProductName=TEP Library
  Subsystem1 : Subsystem
  mmBtu/hr : Product
  tag scope: BM5=global, Q5=global
  wires:
  Exergy1/1 -> Subsystem/1  "Bch5"
  Exergy1/2 -> Subsystem/2  "Bph5"
  Subsystem/1 -> Bus Creator3/1  "Bchm5"
  Subsystem/2 -> Bus Creator3/2  "Bphm5"
  Bus Creator3/1 -> [BM5]  "BM5"
  J/s/1 -> [Q5]
  mmBtu/hr/1 -> J/s/1
  SMEAS 5/1 -> Subsystem1/1(SMEASX)
  [PropertiesStream5] -> Bus Selector2/1
  Subsystem1/1(SMEASXOut) -> Bus Selector1/1
  Bus Selector2/1 -> mmBtu/hr/2  "<HST(5)>"
  Bus Selector2/2 -> Exergy1/1  "<Phase>"
  Bus Selector1/1 -> Exergy1/2  "<SMEAST>"
  Bus Selector1/2 -> Exergy1/4  "<SMEASP>"
  Bus Selector1/3 -> Subsystem/3, mmBtu/hr/1  "<SMEASF>"
  Bus Selector1/4 -> Exergy1/3  "<SMEASX>"

== system TEP_Final_NoScript/Subsystem1/Subsystem5 ==
  SMEAS 13 : Inport
  Bus Creator3 : BusCreator  Inputs=2
  Bus Selector1 : BusSelector  OutputSignals=SMEAST,SMEASP,SMEASF,SMEASX
  Bus Selector2 : BusSelector  OutputSignals=HST(13),Phase
  Exergy1 : mylib/Exergy  SystemSampleTime=-1  VariantActivationTime=update diagram  AllowFlexibleInterface=on  Latency=0  AutoFrameSizeCalculation=off
      settings: SourceProductName=TEP Library
  J/s : Gain  Gain=0.29307107e6
  Subsystem : mylib/Subsystem  SystemSampleTime=-1  VariantActivationTime=update diagram  AllowFlexibleInterface=on  Latency=0  AutoFrameSizeCalculation=off
      settings: SourceProductName=TEP Library
  Subsystem1 : Subsystem
  mmBtu/hr : Product
  tag scope: BM13=global, Q13=global
  wires:
  Exergy1/1 -> Subsystem/1  "Bch13"
  Exergy1/2 -> Subsystem/2  "Bph13"
  Subsystem/1 -> Bus Creator3/1  "Bchm13"
  Subsystem/2 -> Bus Creator3/2  "Bphm13"
  Bus Creator3/1 -> [BM13]  "BM13"
  J/s/1 -> [Q13]
  mmBtu/hr/1 -> J/s/1
  [PropertiesStream13] -> Bus Selector2/1
  SMEAS 13/1 -> Subsystem1/1(SMEASX)
  Subsystem1/1(SMEASXOut) -> Bus Selector1/1
  Bus Selector2/1 -> mmBtu/hr/2  "<HST(13)>"
  Bus Selector2/2 -> Exergy1/1  "<Phase>"
  Bus Selector1/1 -> Exergy1/2  "<SMEAST>"
  Bus Selector1/2 -> Exergy1/4  "<SMEASP>"
  Bus Selector1/3 -> Subsystem/3, mmBtu/hr/1  "<SMEASF>"
  Bus Selector1/4 -> Exergy1/3  "<SMEASX>"

== system TEP_Final_NoScript/Subsystem1/Subsystem6 ==
  Bus Creator : BusCreator  Inputs=15
  SM : Outport  VectorParamsAs1DForOutWhenUnconnected=off
  wires:
  Bus Creator/1 -> SM/1
  [SMCC1] -> Bus Creator/14
  [SM11] -> Bus Creator/10
  [SM5] -> Bus Creator/5
  [SM1] -> Bus Creator/1
  [SM6] -> Bus Creator/6
  [SM9] -> Bus Creator/8
  [SM3] -> Bus Creator/3
  [SM4] -> Bus Creator/4
  [SM10] -> Bus Creator/9
  [SMRC1] -> Bus Creator/12
  [SM2] -> Bus Creator/2
  [SM13] -> Bus Creator/11
  [SM8] -> Bus Creator/7
  [SMRC2] -> Bus Creator/13
  [SMCC2] -> Bus Creator/15

== system TEP_Final_NoScript/Subsystem1/Subsystem8 ==
  SMEAS 1 : Inport
  Bus Creator3 : BusCreator  Inputs=2
  Bus Selector1 : BusSelector  OutputSignals=SMEAST,SMEASP,SMEASF,SMEASX
  Bus Selector2 : BusSelector  OutputSignals=HST(1)
  Exergy1 : mylib/Exergy  SystemSampleTime=-1  VariantActivationTime=update diagram  AllowFlexibleInterface=on  Latency=0  AutoFrameSizeCalculation=off
      settings: SourceProductName=TEP Library
  ITY : Constant
  J/s : Gain  Gain=0.29307107e6
  Subsystem : mylib/Subsystem  SystemSampleTime=-1  VariantActivationTime=update diagram  AllowFlexibleInterface=on  Latency=0  AutoFrameSizeCalculation=off
      settings: SourceProductName=TEP Library
  Subsystem1 : Subsystem
  mmBtu/hr : Product
  tag scope: BM1=global, Q1=global
  wires:
  Exergy1/1 -> Subsystem/1  "Bch1"
  Exergy1/2 -> Subsystem/2  "Bph1"
  Subsystem/1 -> Bus Creator3/1  "Bchm1"
  Subsystem/2 -> Bus Creator3/2  "Bphm1"
  Bus Creator3/1 -> [BM1]  "BM1"
  ITY/1 -> Exergy1/1
  J/s/1 -> [Q1]
  mmBtu/hr/1 -> J/s/1
  SMEAS 1/1 -> Subsystem1/1(SMEASX)
  [PropertiesStream1] -> Bus Selector2/1
  Subsystem1/1(SMEASXOut) -> Bus Selector1/1
  Bus Selector1/1 -> Exergy1/2  "<SMEAST>"
  Bus Selector1/2 -> Exergy1/4  "<SMEASP>"
  Bus Selector1/3 -> mmBtu/hr/1, Subsystem/3  "<SMEASF>"
  Bus Selector1/4 -> Exergy1/3  "<SMEASX>"
  Bus Selector2/1 -> mmBtu/hr/2  "<HST(1)>"

== system TEP_Final_NoScript/Valve/FTM(1) Total molar flow of Stream 1 lb-mol//h ==
  VPOS(1) : Inport
  VRNG(1) : Inport  Port=2
  " " : Product  Inputs=**/
  Constant : Constant  Value=100
  FTM(1) : Outport  PortDimensions=1  VectorParamsAs1DForOutWhenUnconnected=off
  wires:
  VRNG(1)/1 -> " "/2
  Constant/1 -> " "/3
  VPOS(1)/1 -> " "/1
  " "/1 -> FTM(1)/1

== system TEP_Final_NoScript/Valve/Position of Valve 1 % ==
  Bus Selector : BusSelector  OutputSignals=XMV(1)
  Control valve : mylib/Control valve  SystemSampleTime=-1  VariantActivationTime=update diagram  AllowFlexibleInterface=on  Latency=0  AutoFrameSizeCalculation=off
      settings: SourceProductName=TEP Library
  Display : Display
  Divide : Product  Inputs=*/
  IVST(1) : Constant  Value=0
  Integration : mylib/Integration  SystemSampleTime=-1  VariantActivationTime=update diagram  AllowFlexibleInterface=on  Latency=0  AutoFrameSizeCalculation=off
      settings: SourceProductName=TEP Library
  Subtract : Sum  Inputs=+-
  VTAU(1) : Constant  Value=8/3600
  YY(39) : Constant  Value=63.05263039
  "YY(39) " : Outport  VectorParamsAs1DForOutWhenUnconnected=off
  wires:
  Integration/1 -> "YY(39) "/1, Subtract/2  "VPOS(1)"
  YY(39)/1 -> Integration/2
  Subtract/1 -> Divide/1
  VTAU(1)/1 -> Divide/2
  Divide/1 -> Display/1, Integration/1
  Control valve/1 -> Subtract/1
  [XMV] -> Bus Selector/1
  Bus Selector/1 -> Control valve/1  "<XMV(1)>"
  IVST(1)/1 -> Control valve/2

== system TEP_Final_NoScript/Valve 2/FTM(2) Total molar flow of Stream 2 lb-mol//h ==
  VPOS(2) : Inport
  VRNG(2) : Inport  Port=2
  " " : Product  Inputs=**/
  Constant : Constant  Value=100
  FTM(2) : Outport  PortDimensions=1  VectorParamsAs1DForOutWhenUnconnected=off
  wires:
  VRNG(2)/1 -> " "/2
  Constant/1 -> " "/3
  VPOS(2)/1 -> " "/1
  " "/1 -> FTM(2)/1

== system TEP_Final_NoScript/Valve 2/Position of Valve 2 % ==
  Bus Selector : BusSelector  OutputSignals=XMV(2)
  Control valve : mylib/Control valve  SystemSampleTime=-1  VariantActivationTime=update diagram  AllowFlexibleInterface=on  Latency=0  AutoFrameSizeCalculation=off
      settings: SourceProductName=TEP Library
  Divide : Product  Inputs=*/
  IVST(2) : Constant  Value=0
  Integration : mylib/Integration  SystemSampleTime=-1  VariantActivationTime=update diagram  AllowFlexibleInterface=on  Latency=0  AutoFrameSizeCalculation=off
      settings: SourceProductName=TEP Library
  Subtract : Sum  Inputs=+-
  VTAU(2) : Constant  Value=8/3600
  YY(40) : Constant  Value=53.97970677
  "YY(40)  " : Outport  VectorParamsAs1DForOutWhenUnconnected=off
  wires:
  Control valve/1 -> Subtract/1
  Subtract/1 -> Divide/1
  VTAU(2)/1 -> Divide/2
  Divide/1 -> Integration/1
  Integration/1 -> Subtract/2, "YY(40)  "/1  "VPOS(2)"
  YY(40)/1 -> Integration/2
  [XMV] -> Bus Selector/1
  Bus Selector/1 -> Control valve/1  "<XMV(2)>"
  IVST(2)/1 -> Control valve/2

== system TEP_Final_NoScript/Valve 3/FTM(3) Total molar flow of Stream 3 lb-mol//h ==
  VPOS(3) : Inport
  VRNG(3) : Inport  Port=2
  " " : Product  Inputs=***/
  Bus Selector : BusSelector  OutputSignals=IDV(6)
  Constant : Constant  Value=100
  Constant1 : Constant
  Subtract : Sum  Inputs=+-
  FTM(3) : Outport  PortDimensions=1  VectorParamsAs1DForOutWhenUnconnected=off
  wires:
  VPOS(3)/1 -> " "/1
  " "/1 -> FTM(3)/1
  Constant1/1 -> Subtract/1
  [IDV] -> Bus Selector/1
  Constant/1 -> " "/4
  Subtract/1 -> " "/2
  VRNG(3)/1 -> " "/3
  Bus Selector/1 -> Subtract/2  "<IDV(6)>"

== system TEP_Final_NoScript/Valve 3/Position of Valve 3 % ==
  Bus Selector : BusSelector  OutputSignals=XMV(3)
  Control valve : mylib/Control valve  SystemSampleTime=-1  VariantActivationTime=update diagram  AllowFlexibleInterface=on  Latency=0  AutoFrameSizeCalculation=off
      settings: SourceProductName=TEP Library
  Divide : Product  Inputs=*/
  IVST(3) : Constant  Value=0
  Integration : mylib/Integration  SystemSampleTime=-1  VariantActivationTime=update diagram  AllowFlexibleInterface=on  Latency=0  AutoFrameSizeCalculation=off
      settings: SourceProductName=TEP Library
  Subtract : Sum  Inputs=+-
  VTAU(3) : Constant  Value=6/3600
  YY(41) : Constant  Value=24.64355755
  "YY(41) " : Outport  VectorParamsAs1DForOutWhenUnconnected=off
  wires:
  Control valve/1 -> Subtract/1
  Subtract/1 -> Divide/1
  VTAU(3)/1 -> Divide/2
  Divide/1 -> Integration/1
  Integration/1 -> "YY(41) "/1, Subtract/2  "VPOS(3)"
  YY(41)/1 -> Integration/2
  [XMV] -> Bus Selector/1
  Bus Selector/1 -> Control valve/1  "<XMV(3)>"
  IVST(3)/1 -> Control valve/2

== system TEP_Final_NoScript/Valve 4/FTM(4) Total molar flow of Stream 4 lb-mol//h ==
  VPOS(4) : Inport
  VRNG(4) : Inport  Port=2
  " " : Product  Inputs=***/
  Add : Sum
  Bus Selector : BusSelector  OutputSignals=IDV(7)
  Constant : Constant
  Constant1 : Constant  Value=0.2
  Constant3 : Constant  Value=100
  Constant4 : Constant  Value=1e-10
  Product1 : Product
  Subtract : Sum  Inputs=+-
  FTM(4) : Outport  PortDimensions=1  VectorParamsAs1DForOutWhenUnconnected=off
  wires:
  Add/1 -> FTM(4)/1
  Constant4/1 -> Add/2
  " "/1 -> Add/1
  VPOS(4)/1 -> " "/1
  Bus Selector/1 -> Product1/1  "<IDV(7)>"
  Product1/1 -> Subtract/2
  Constant1/1 -> Product1/2
  Constant/1 -> Subtract/1
  Constant3/1 -> " "/4
  VRNG(4)/1 -> " "/3
  Subtract/1 -> " "/2
  [IDV] -> Bus Selector/1

== system TEP_Final_NoScript/Valve 4/Position of Valve 4 % ==
  Bus Selector : BusSelector  OutputSignals=XMV(4)
  Control valve : mylib/Control valve  SystemSampleTime=-1  VariantActivationTime=update diagram  AllowFlexibleInterface=on  Latency=0  AutoFrameSizeCalculation=off
      settings: SourceProductName=TEP Library
  Divide : Product  Inputs=*/
  IVST(4) : Constant  Value=0
  Integration : mylib/Integration  SystemSampleTime=-1  VariantActivationTime=update diagram  AllowFlexibleInterface=on  Latency=0  AutoFrameSizeCalculation=off
      settings: SourceProductName=TEP Library
  Subtract : Sum  Inputs=+-
  VTAU(4) : Constant  Value=9/3600
  YY(42) : Constant  Value=61.30192144
  "YY(42) " : Outport  VectorParamsAs1DForOutWhenUnconnected=off
  wires:
  Control valve/1 -> Subtract/1
  Subtract/1 -> Divide/1
  VTAU(4)/1 -> Divide/2
  Divide/1 -> Integration/1
  Integration/1 -> "YY(42) "/1, Subtract/2  "VPOS(4)"
  YY(42)/1 -> Integration/2
  [XMV] -> Bus Selector/1
  Bus Selector/1 -> Control valve/1  "<XMV(4)>"
  IVST(4)/1 -> Control valve/2

== system TEP_Final_NoScript/Compressor/Subsystem/If Action Subsystem ==
  In1 : Inport
  Action Port : ActionPort  ActionPortLabel=if(u1 < 1)
  Out1 : Outport  VectorParamsAs1DForOutWhenUnconnected=off
  wires:
  In1/1 -> Out1/1

== system TEP_Final_NoScript/Compressor/Subsystem/If Action Subsystem1 ==
  In1 : Inport
  Action Port : ActionPort  ActionPortLabel=elseif(u1>1.3)
  Out1 : Outport  VectorParamsAs1DForOutWhenUnconnected=off
  wires:
  In1/1 -> Out1/1

== system TEP_Final_NoScript/Compressor/Subsystem/If Action Subsystem2 ==
  In1 : Inport
  Action Port : ActionPort  ActionPortLabel=else
  Out1 : Outport  VectorParamsAs1DForOutWhenUnconnected=off
  wires:
  In1/1 -> Out1/1

== system TEP_Final_NoScript/Condenser/Cooling water outlet temperature/TCWS Inlet temperature of cooling water °C ==
  Add : Sum
  Bus Selector : BusSelector  OutputSignals=signal1.TESUB8(6)
  Bus Selector1 : BusSelector  OutputSignals=IDV(5)
  Constant : Constant  Value=5
  Product1 : Product
  TCWS : Outport  VectorParamsAs1DForOutWhenUnconnected=off
  wires:
  Constant/1 -> Product1/2
  Bus Selector/1 -> Add/1  "<TESUB8(6)>"
  Bus Selector1/1 -> Product1/1  "<IDV(5)>"
  [TESUB8] -> Bus Selector/1
  Product1/1 -> Add/2
  [IDV] -> Bus Selector1/1
  Add/1 -> TCWS/1

== system TEP_Final_NoScript/Mixing Zone/Holdup of Components in Mixing Zone/Holdup of Vapour Components in the Mixing Zone ==
  YY(28:35) : Inport
  Bus Creator : BusCreator  Inputs=8
  Bus Selector4 : BusSelector  OutputSignals=YY(28),YY(29),YY(30),YY(31),YY(32),YY(33),YY(34),YY(35)
  UCVV(1) Holdup of Component A (Vapour) in Mixing zone lb-mol : Gain
  UCVV(2) Holdup of Component B (Vapour) in Mixing zone lb-mol : Gain
  UCVV(3) Holdup of Component C (Vapour) in Mixing zone lb-mol : Gain
  UCVV(4) Holdup of Component D (Vapour) in Mixing zone lb-mol : Gain
  UCVV(5) Holdup of Component E (Vapour) in Mixing zone lb-mol : Gain
  UCVV(6) Holdup of Component F (Vapour) in Mixing zone lb-mol : Gain
  UCVV(7) Holdup of Component G (Vapour) in Mixing zone lb-mol : Gain
  UCVV(8) Holdup of Component H (Vapour) in Mixing zone lb-mol : Gain
  UCVV : Outport  VectorParamsAs1DForOutWhenUnconnected=off
  wires:
  Bus Selector4/7 -> UCVV(7) Holdup of Component G (Vapour) in Mixing zone lb-mol/1  "<YY(34)>"
  Bus Selector4/2 -> UCVV(2) Holdup of Component B (Vapour) in Mixing zone lb-mol/1  "<YY(29)>"
  Bus Selector4/3 -> UCVV(3) Holdup of Component C (Vapour) in Mixing zone lb-mol/1  "<YY(30)>"
  Bus Selector4/4 -> UCVV(4) Holdup of Component D (Vapour) in Mixing zone lb-mol/1  "<YY(31)>"
  Bus Selector4/5 -> UCVV(5) Holdup of Component E (Vapour) in Mixing zone lb-mol/1  "<YY(32)>"
  Bus Selector4/6 -> UCVV(6) Holdup of Component F (Vapour) in Mixing zone lb-mol/1  "<YY(33)>"
  Bus Selector4/1 -> UCVV(1) Holdup of Component A (Vapour) in Mixing zone lb-mol/1  "<YY(28)>"
  Bus Selector4/8 -> UCVV(8) Holdup of Component H (Vapour) in Mixing zone lb-mol/1  "<YY(35)>"
  YY(28:35)/1 -> Bus Selector4/1
  UCVV(1) Holdup of Component A (Vapour) in Mixing zone lb-mol/1 -> Bus Creator/1  "UCVV(1)"
  UCVV(2) Holdup of Component B (Vapour) in Mixing zone lb-mol/1 -> Bus Creator/2  "UCVV(2)"
  UCVV(3) Holdup of Component C (Vapour) in Mixing zone lb-mol/1 -> Bus Creator/3  "UCVV(3)"
  UCVV(4) Holdup of Component D (Vapour) in Mixing zone lb-mol/1 -> Bus Creator/4  "UCVV(4)"
  UCVV(5) Holdup of Component E (Vapour) in Mixing zone lb-mol/1 -> Bus Creator/5  "UCVV(5)"
  UCVV(6) Holdup of Component F (Vapour) in Mixing zone lb-mol/1 -> Bus Creator/6  "UCVV(6)"
  UCVV(7) Holdup of Component G (Vapour) in Mixing zone lb-mol/1 -> Bus Creator/7  "UCVV(7)"
  UCVV(8) Holdup of Component H (Vapour) in Mixing zone lb-mol/1 -> Bus Creator/8  "UCVV(8)"
  Bus Creator/1 -> UCVV/1
